simulink model "proiectFCC"  (R2020b)
settings: Solver=VariableStepAuto  StartTime=0.0  StopTime=10.0  RelTol=1e-3
undefined symbols (not defined in the file): A, a0, a1, a2, a3, B, b10, b11, b12, C, D, den, num
settings Model: Creator=Alex  LastModifiedBy=Alex

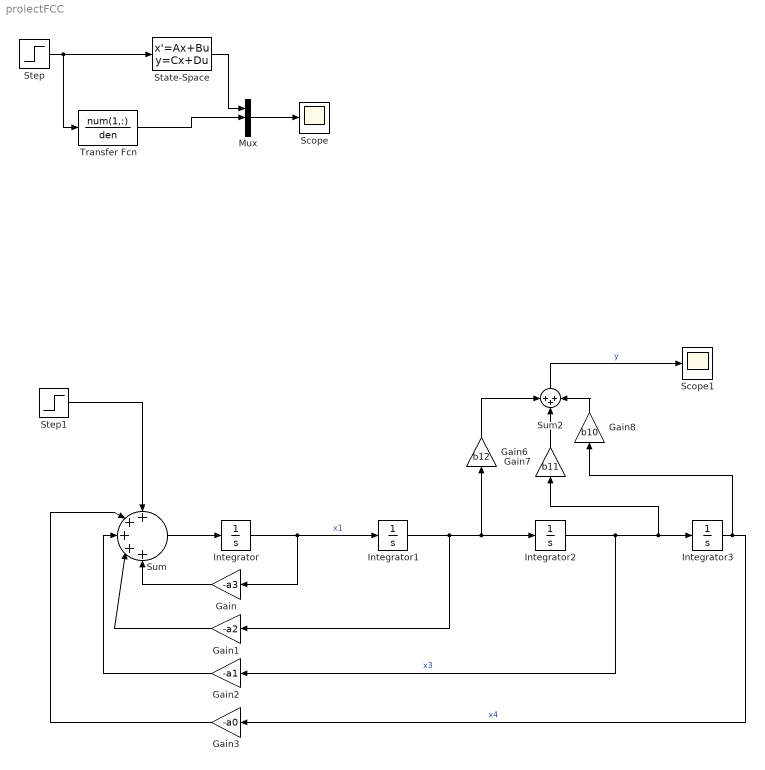
== system proiectFCC ==
  Gain : Gain  Gain=-a3
  Gain1 : Gain  Gain=-a2
  Gain2 : Gain  Gain=-a1
  Gain3 : Gain  Gain=-a0
  Gain6 : Gain  Gain=b12
  Gain7 : Gain  Gain=b11
  Gain8 : Gain  Gain=b10
  Integrator{,1..3} (4 alike) : Integrator
  Mux : Mux  Inputs=3
  Scope : Scope
  Scope1 : Scope
  State-Space : StateSpace  A=A  B=B  C=C  D=D  InitialCondition=0
  Step : Step  SampleTime=0
  Step1 : Step  SampleTime=0
  Sum : Sum  Inputs=+|+|+|+|+
  Sum2 : Sum  Inputs=+++
  Transfer Fcn : TransferFcn  Numerator=num(1,:)  Denominator=den
  wires:
  Step/1 -> Transfer Fcn/1, State-Space/1
  Mux/1 -> Scope/1
  State-Space/1 -> Mux/1
  Transfer Fcn/1 -> Mux/2
  Integrator2/1 -> Gain2/1, Gain7/1, Integrator3/1  "x3"
  Integrator3/1 -> Gain3/1, Gain8/1  "x4"
  Integrator1/1 -> Gain1/1, Gain6/1, Integrator2/1
  Integrator/1 -> Gain/1, Integrator1/1  "x1"
  Gain/1 -> Sum/5
  Gain1/1 -> Sum/4
  Gain2/1 -> Sum/3
  Step1/1 -> Sum/1
  Sum/1 -> Integrator/1
  Gain3/1 -> Sum/2
  Gain6/1 -> Sum2/1
  Gain7/1 -> Sum2/2
  Gain8/1 -> Sum2/3
  Sum2/1 -> Scope1/1  "y"
